simulink model "BatteryPack"  (R2023b)
settings: Solver=VariableStepAuto  StartTime=0.0  StopTime=10.0  RelTol=1e-3
InitFcn:
  | eta=0.992943452611046;
  | Q=5.134436834270520;
  | Qinv=1/Q;
  | Qinv_cells=Qinv+0.01*rand(12,1);
  | delta_t=0.1;
  | delta_t_delta=4;
  | taw=2.410723815561624;
  | R0=0.011163238296886;
  | R0_cells=R0+0.001*rand(12,1);
  | R=0.002515135572506;
  | gamma=61.749752200480295;
  | M0=0.002542395121461;
  | M=0.044341699418566;
  | OCV0=[3.03083668947220,3.16996176507765,3.24654613672245,3.30462471088150,3.35178831826018,3.39207985837564,3.42754280925954,3.45930893308633,3.48845834377828,3.51506471884948,3.53941528250350,3.56229005089512,3.58347680139773,3.60345371361795,3.62204667414497,3.63945293994712,3.65555208129593,3.67025842747189,3.68283722926942,3.69256635796299,3.69934356504319,3.70421492193387,3.70864080668278,3.71251647816700,3.71676450243010,3.72076080442289,3.72459036631361,3.72852113964889,3.73262555664002,3.73679788031633,3.74085805813141,3.74504293170943,3.74937151420852,3.75360503345497,3.75808554938499,3.76253512812700,3.76686713224277,3.77129741354356,3.77568299945893,3.78010899552110,3.78432597237866,3.78866667245794,3.79282973590265,3.79699149175738,3.80102646886227,3.80486901671467,3.80859160652083,3.81234290326678,3.81578374146922,3.81901029060391,3.82246264968075,3.82565270541301,3.82878492908885,3.83182846251259,3.83504605065465,3.83817152994830,3.84120926637331,3.84427045104513,3.84745505461551,3.85048527227548,3.85338258086535,3.85633375142700,3.85903736950342,3.86183294078638,3.86426909473005,3.86668409269911,3.86884960464201,3.87075062579497,3.87260151166861,3.87419873493045,3.87590354579771,3.87742660309802,3.87888623494178,3.88013778482297,3.88172955555187,3.88298517380087,3.88445139467736,3.88588841874555,3.88718906620625,3.88865483707461,3.89034900018679,3.89177308296385,3.89345014882802,3.89492324307466,3.89656804158261,3.89814831273987,3.89970800088682,3.90138268502894,3.90325919869100,3.90466035566401,3.90650715226313,3.90818394205928,3.90991726595604,3.91178869314647,3.91353048350435,3.91535717290223,3.91722943087205,3.91902077537227,3.92094773764149,3.92272669049051,3.92480210727778,3.92665898861166,3.92855163124444,3.93049425931182,3.93233822864100,3.93413808807444,3.93586787406902,3.93781878301823,3.93970352375448,3.94141217835583,3.94337738846496,3.94524781610469,3.94705512196599,3.94889596931986,3.95072813117993,3.95268786149774,3.95437483545637,3.95614043217004,3.95813802002780,3.95988737276266,3.96180145819164,3.96333094922522,3.96513598465409,3.96688905019200,3.96847526303094,3.97032227257873,3.97189764460202,3.97357890138617,3.97507568580842,3.97666308363629,3.97834004990894,3.97972757215233,3.98134719919954,3.98282452838428,3.98434240750033,3.98579080664983,3.98712095624815,3.98848186479248,3.99005169119157,3.99140961007081,3.99272279272243,3.99405266719970,3.99553040552875,3.99686295933407,3.99826042332052,3.99959085613132,4.00118770124588,4.00258756750194,4.00410831223298,4.00564378913664,4.00733579962478,4.00874100440808,4.01049664802522,4.01229894715480,4.01403904622199,4.01578258632489,4.01777261837808,4.01971351876421,4.02181419747090,4.02405411757281,4.02634132187682,4.02844966043338,4.03074821161091,4.03287252710406,4.03519979075052,4.03714724603729,4.03920059502787,4.04119005170582,4.04311251958802,4.04485629277420,4.04687276700581,4.04856655229106,4.05028282064349,4.05188790780758,4.05367115501827,4.05540888556017,4.05715082708000,4.05891707849673,4.06058066558082,4.06255984784218,4.06443355862160,4.06646437679668,4.06828978114252,4.07040446117501,4.07260180541029,4.07472443659757,4.07695226365058,4.07952388568996,4.08211497603818,4.08494517654941,4.08785760361077,4.09108975271414,4.09441257923899,4.09808703497329,4.10213358582538,4.10639223642507,4.11114147862302,4.11656968526475,4.12276605724301,4.13028542232852,4.14480757713318];
  | OCVrel=[-0.000420362949371303,-0.000578339102606499,-0.000548212633161139,-0.000532050376255593,-0.000513855468461292,-0.000495687320522634,-0.000487643250941371,-0.000470920985950642,-0.000461928451583620,-0.000448574992511236,-0.000430345291794665,-0.000415864789930715,-0.000403503275736067,-0.000392608506451838,-0.000381149699535297,-0.000369136346590911,-0.000348156127830507,-0.000324184515919599,-0.000280229092973681,-0.000201932662233446,-0.000110744926726894,-3.79084757376537e-05,7.34820416665105e-08,1.98249344364182e-05,1.89028531032423e-05,1.52778169972465e-05,1.34924868477160e-05,9.23542420261725e-06,-1.46245586440975e-06,-1.45311365618779e-05,-2.47366010229282e-05,-3.53430095058658e-05,-4.35761509840300e-05,-4.95443607046995e-05,-5.59569418266839e-05,-5.71405250985218e-05,-5.58628466608733e-05,-5.23710248925624e-05,-5.22024906444821e-05,-5.10066281299635e-05,-4.60070072284917e-05,-4.39210588487260e-05,-4.17087376582674e-05,-3.79965319780425e-05,-3.52883378328963e-05,-2.96358522826692e-05,-1.93487210265394e-05,-1.76654799578108e-05,-1.10481636980021e-05,-6.29033346947879e-06,-6.43729682754031e-06,-8.99082338466702e-06,-5.97476480532998e-06,-4.62198779734926e-06,-8.45626888598137e-06,-3.55310580626464e-06,1.21105779784145e-06,3.23270957394308e-06,4.65975925632772e-06,6.06047576788568e-06,1.06741421249725e-05,1.27740668978125e-05,1.58322240631086e-05,1.58226143080902e-05,1.77356396535024e-05,1.67297263145319e-05,2.20422014608934e-05,3.24455524629346e-05,4.53671310943400e-05,6.36631547519500e-05,7.65783816690908e-05,9.78737779086299e-05,0.000118072210378981,0.000145052733908454,0.000159053964033644,0.000178615115542580,0.000192951944721033,0.000203745870809340,0.000215887472157157,0.000217389449254637,0.000214080259255523,0.000217368801393146,0.000210680488604522,0.000216791472310507,0.000210807141665482,0.000206892775031066,0.000209889448971827,0.000206480366569060,0.000197477832361696,0.000201878205171392,0.000195991461516702,0.000193299624131949,0.000189225295900371,0.000183015755985024,0.000181030375137689,0.000179058026812520,0.000172630244233569,0.000169739554492468,0.000168470860940041,0.000165673583835095,0.000158761613569570,0.000158310548246597,0.000160768730786868,0.000159274891317150,0.000163654237071923,0.000165646854650985,0.000171009006229332,0.000172960872040281,0.000174059186593325,0.000184792008315373,0.000185457536514424,0.000188497928404933,0.000193540560057086,0.000201967121634793,0.000208651810099923,0.000210203310502306,0.000221327742354831,0.000226934798568295,0.000229022527795167,0.000235980838038274,0.000237393722897026,0.000251416377586933,0.000255669183930939,0.000259582507624291,0.000271756110286130,0.000271428141354407,0.000280338423121521,0.000282159563486788,0.000293698306662556,0.000294690382734668,0.000296368480075595,0.000305852381154249,0.000305547730725772,0.000310124564075650,0.000308910141248888,0.000310910207998593,0.000317136879477080,0.000319966110029179,0.000317781933009713,0.000319714895363342,0.000323633211007860,0.000324670146330631,0.000321258389806546,0.000325090635960723,0.000325756317802870,0.000329299487485483,0.000323022114762843,0.000329687741218402,0.000331335077114761,0.000334366863810491,0.000334190313302610,0.000348244516476559,0.000353619969496185,0.000370645612717080,0.000387424759796793,0.000412712601107454,0.000432980002313212,0.000458081645703528,0.000475316126710853,0.000488710969037302,0.000490229811285922,0.000496997034255361,0.000490732502998424,0.000485413024014050,0.000470031399074122,0.000464225038785084,0.000453594366571016,0.000442947689735187,0.000432361194051228,0.000426870028472560,0.000412534978795853,0.000404144406879032,0.000399500637103100,0.000395361789641937,0.000391903989806764,0.000388094198725783,0.000384493593513828,0.000380890719331740,0.000381944387481867,0.000375725748044827,0.000377689116895975,0.000371263292977880,0.000375401761542324,0.000371961214504098,0.000372140497419301,0.000376623010739057,0.000379713082469440,0.000373305112977953,0.000376271071938692,0.000374048457576144,0.000373866132643822,0.000368451986163444,0.000366513632840686,0.000361449855405437,0.000355758001511034,0.000351852945592445,0.000340424192937049,0.000323803410913197,0.000299570003101876,0.000255297108741397,9.12380218506306e-05];
  | soc_values=[0,0.00500000000000000,0.0100000000000000,0.0150000000000000,0.0200000000000000,0.0250000000000000,0.0300000000000000,0.0350000000000000,0.0400000000000000,0.0450000000000000,0.0500000000000000,0.0550000000000000,0.0600000000000000,0.0650000000000000,0.0700000000000000,0.0750000000000000,0.0800000000000000,0.0850000000000000,0.0900000000000000,0.0950000000000000,0.100000000000000,0.105000000000000,0.110000000000000,0.115000000000000,0.120000000000000,0.125000000000000,0.130000000000000,0.135000000000000,0.140000000000000,0.145000000000000,0.150000000000000,0.155000000000000,0.160000000000000,0.165000000000000,0.170000000000000,0.175000000000000,0.180000000000000,0.185000000000000,0.190000000000000,0.195000000000000,0.200000000000000,0.205000000000000,0.210000000000000,0.215000000000000,0.220000000000000,0.225000000000000,0.230000000000000,0.235000000000000,0.240000000000000,0.245000000000000,0.250000000000000,0.255000000000000,0.260000000000000,0.265000000000000,0.270000000000000,0.275000000000000,0.280000000000000,0.285000000000000,0.290000000000000,0.295000000000000,0.300000000000000,0.305000000000000,0.310000000000000,0.315000000000000,0.320000000000000,0.325000000000000,0.330000000000000,0.335000000000000,0.340000000000000,0.345000000000000,0.350000000000000,0.355000000000000,0.360000000000000,0.365000000000000,0.370000000000000,0.375000000000000,0.380000000000000,0.385000000000000,0.390000000000000,0.395000000000000,0.400000000000000,0.405000000000000,0.410000000000000,0.415000000000000,0.420000000000000,0.425000000000000,0.430000000000000,0.435000000000000,0.440000000000000,0.445000000000000,0.450000000000000,0.455000000000000,0.460000000000000,0.465000000000000,0.470000000000000,0.475000000000000,0.480000000000000,0.485000000000000,0.490000000000000,0.495000000000000,0.500000000000000,0.505000000000000,0.510000000000000,0.515000000000000,0.520000000000000,0.525000000000000,0.530000000000000,0.535000000000000,0.540000000000000,0.545000000000000,0.550000000000000,0.555000000000000,0.560000000000000,0.565000000000000,0.570000000000000,0.575000000000000,0.580000000000000,0.585000000000000,0.590000000000000,0.595000000000000,0.600000000000000,0.605000000000000,0.610000000000000,0.615000000000000,0.620000000000000,0.625000000000000,0.630000000000000,0.635000000000000,0.640000000000000,0.645000000000000,0.650000000000000,0.655000000000000,0.660000000000000,0.665000000000000,0.670000000000000,0.675000000000000,0.680000000000000,0.685000000000000,0.690000000000000,0.695000000000000,0.700000000000000,0.705000000000000,0.710000000000000,0.715000000000000,0.720000000000000,0.725000000000000,0.730000000000000,0.735000000000000,0.740000000000000,0.745000000000000,0.750000000000000,0.755000000000000,0.760000000000000,0.765000000000000,0.770000000000000,0.775000000000000,0.780000000000000,0.785000000000000,0.790000000000000,0.795000000000000,0.800000000000000,0.805000000000000,0.810000000000000,0.815000000000000,0.820000000000000,0.825000000000000,0.830000000000000,0.835000000000000,0.840000000000000,0.845000000000000,0.850000000000000,0.855000000000000,0.860000000000000,0.865000000000000,0.870000000000000,0.875000000000000,0.880000000000000,0.885000000000000,0.890000000000000,0.895000000000000,0.900000000000000,0.905000000000000,0.910000000000000,0.915000000000000,0.920000000000000,0.925000000000000,0.930000000000000,0.935000000000000,0.940000000000000,0.945000000000000,0.950000000000000,0.955000000000000,0.960000000000000,0.965000000000000,0.970000000000000,0.975000000000000,0.980000000000000,0.985000000000000,0.990000000000000,0.995000000000000,1];
  | OCV_values=OCV0+25*OCVrel;
  | dZ = soc_values(2) - soc_values(1); % Find spacing of SOC vector
  | dUdZ = diff(OCV_values)/dZ; % Scaled forward finite difference
  | dOCV = ([dUdZ(1) dUdZ] + [dUdZ dUdZ(end)])/2; % Avg of fwd/bkwd diffs
  | SigmaX0 = diag([1e-3 1e-3 1e-2]); % uncertainty of initial state
  | sigmaV = 2e-1; % uncertainty of voltage sensor, output equation
  | sigmaW = 1e1; % uncertainty of current sensor, state equation
  | vbar=0;
  | w_bar=0;
  | nR=0.004;
  | nQ=0.05;
  | ek=0.01;
  | Vmax=4.2;
  | Vmin=2.7;
  | Imax=2*Q;
  | Standby=0;
  | Charging=1;
  | Discharging=2;
  | load('BattCrntDrvCycle.mat');
undefined symbols (not defined in the file): AUX0_OV, AUX1_OV, AUX2_OV, AUX3_OV, AUX4_OV, NCHAN
libraries: fl_lib x130, nesl_utility x88, simulink x53, ee_lib x37, batt_lib x36, eeGeneralControl x21, hdlsllib x9
(part 1 of 10)
settings Model: Creator=Alkhouly  LastModifiedBy=Alkhouly

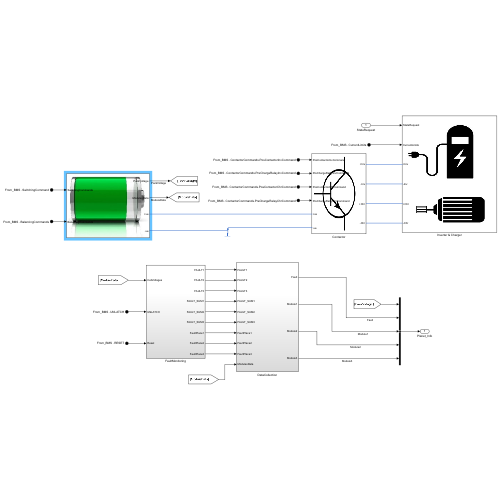
[thumbnail: Simulink's stored preview of the top-level diagram]
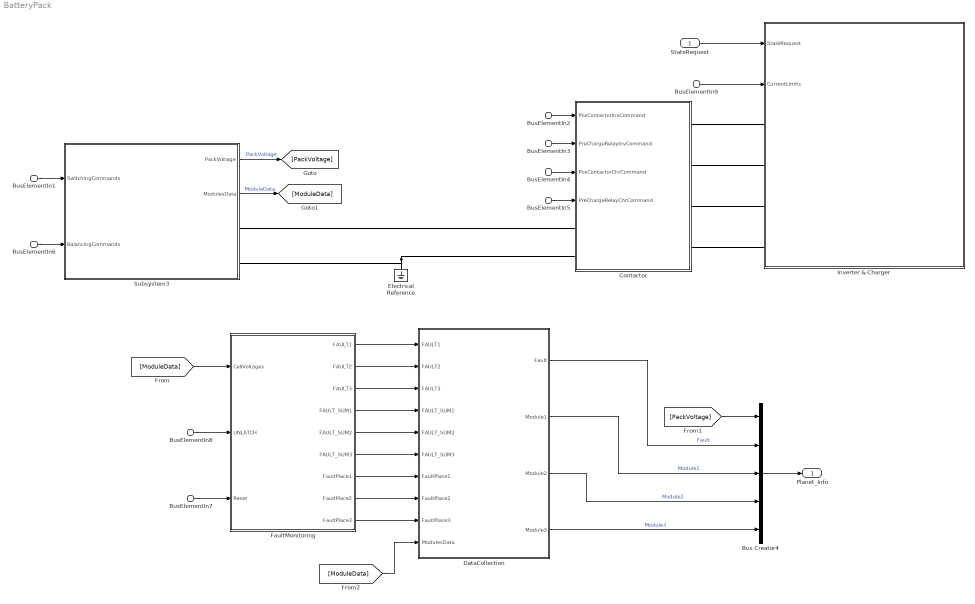
== system BatteryPack ==
  StateRequest : Inport
  BusElementIn2 : Inport  Port=2  PortName=From_BMS  Element=ContactorCommands.PosContactorInvCommand
  BusElementIn3 : Inport  Port=2  PortName=From_BMS  Element=ContactorCommands.PreChargeRelayInvCommand
  BusElementIn4 : Inport  Port=2  PortName=From_BMS  Element=ContactorCommands.PosContactorChrCommand
  BusElementIn5 : Inport  Port=2  PortName=From_BMS  Element=ContactorCommands.PreChargeRelayChrCommand
  BusElementIn1 : Inport  Port=2  PortName=From_BMS  Element=SwitchingCommand
  BusElementIn8 : Inport  Port=2  PortName=From_BMS  Element=UNLATCH
  BusElementIn7 : Inport  Port=2  PortName=From_BMS  Element=RESET
  BusElementIn6 : Inport  Port=2  PortName=From_BMS  Element=BalancingCommands
  BusElementIn9 : Inport  Port=2  PortName=From_BMS  Element=CurrentLimits
  Bus Creator4 : BusCreator  Inputs=5
  Contactor : Subsystem
      mask Display: image('PowerElectronics.jpg');
  DataCollection : Subsystem
  Electrical Reference : fl_lib/Electrical/Electrical Elements/Electrical Reference
  FaultMonitoring : Subsystem
  Inverter & Charger : Subsystem
      mask Display: image('Charger_Load3.jpg');
  Subsystem3 : Subsystem
      mask Display: image('Plant_Battery.jpg');
  Planet_Info : Outport
  wires:
  StateRequest/1 -> Inverter & Charger/1(StateRequest)
  Subsystem3/1(PackVoltage) -> [PackVoltage]  "PackVoltage"
  Subsystem3/2(ModulesData) -> [ModuleData]  "ModuleData"
  [ModuleData] -> FaultMonitoring/1(CellVoltages)
  [PackVoltage] -> Bus Creator4/1
  BusElementIn2/1 -> Contactor/1(PosContactorInvCommand)
  BusElementIn3/1 -> Contactor/2(PreChargeRelayInvCommand)
  BusElementIn4/1 -> Contactor/3(PosContactorChrCommand)
  BusElementIn5/1 -> Contactor/4(PreChargeRelayChrCommand)
  BusElementIn1/1 -> Subsystem3/1(SwitchingCommands)
  BusElementIn6/1 -> Subsystem3/2(BalancingCommands)
  BusElementIn7/1 -> FaultMonitoring/3(Reset)
  BusElementIn8/1 -> FaultMonitoring/2(UNLATCH)
  BusElementIn9/1 -> Inverter & Charger/2(CurrentLimits)
  FaultMonitoring/1(FAULT1) -> DataCollection/1(FAULT1)
  FaultMonitoring/2(FAULT2) -> DataCollection/2(FAULT2)
  FaultMonitoring/3(FAULT3) -> DataCollection/3(FAULT3)
  FaultMonitoring/4(FAULT_SUM1) -> DataCollection/4(FAULT_SUM1)
  FaultMonitoring/5(FAULT_SUM2) -> DataCollection/5(FAULT_SUM2)
  FaultMonitoring/6(FAULT_SUM3) -> DataCollection/6(FAULT_SUM3)
  FaultMonitoring/7(FaultPlace1) -> DataCollection/7(FaultPlace1)
  FaultMonitoring/8(FaultPlace2) -> DataCollection/8(FaultPlace2)
  FaultMonitoring/9(FaultPlace3) -> DataCollection/9(FaultPlace3)
  [ModuleData] -> DataCollection/10(ModulesData)
  DataCollection/1(Fault) -> Bus Creator4/2  "Fault"
  DataCollection/2(Module1) -> Bus Creator4/3  "Module1"
  DataCollection/3(Module2) -> Bus Creator4/4  "Module2"
  DataCollection/4(Module3) -> Bus Creator4/5  "Module3"
  Bus Creator4/1 -> Planet_Info/1
  connections:
  Subsystem3/RConn1 -- Contactor/LConn1
  Contactor/RConn3 -- Inverter & Charger/LConn3
  Contactor/RConn2 -- Inverter & Charger/LConn2
  Contactor/RConn4 -- Inverter & Charger/LConn4
  Contactor/RConn1 -- Inverter & Charger/LConn1
  Subsystem3/RConn2 -- Electrical Reference/LConn1 -- Contactor/LConn2

== system BatteryPack/Contactor ==
  PosContactorInvCommand : Inport
  PreChargeRelayInvCommand : Inport  Port=2
  PosContactorChrCommand : Inport  Port=3
  PreChargeRelayChrCommand : Inport  Port=4
  Capacitor : fl_lib/Electrical/Electrical Elements/Capacitor  c=10000 uF  r=1e-6 Ohm  g=0 1/Ohm  i_specify=off  i_priority=None  i=0 A  i_nominal_specify=off  i_nominal_unit=A  i_nominal_value=1  v_specify=off  v_priority=None  v=0 V  v_nominal_specify=off  v_nominal_unit=V  v_nominal_value=1  vc_specify=off  vc_priority=High  vc=0 V  vc_nominal_specify=off  vc_nominal_unit=V  vc_nominal_value=1
  Capacitor1 : fl_lib/Electrical/Electrical Elements/Capacitor  c=10000 uF  r=1e-6 Ohm  g=0 1/Ohm  i_specify=off  i_priority=None  i=0 A  i_nominal_specify=off  i_nominal_unit=A  i_nominal_value=1  v_specify=off  v_priority=None  v=0 V  v_nominal_specify=off  v_nominal_unit=V  v_nominal_value=1  vc_specify=off  vc_priority=High  vc=0 V  vc_nominal_specify=off  vc_nominal_unit=V  vc_nominal_value=1
  Data Type Conversion{,1,3..4} (4 alike) : DataTypeConversion  SaturateOnIntegerOverflow=off  RndMeth=Floor
  Resistor : fl_lib/Electrical/Electrical Elements/Resistor  R=20 Ohm  i_specify=off  i_priority=None  i=0 A  i_nominal_specify=off  i_nominal_unit=A  i_nominal_value=1  v_specify=off  v_priority=None  v=0 V  v_nominal_specify=off  v_nominal_unit=V  v_nominal_value=1
  Resistor1 : fl_lib/Electrical/Electrical Elements/Resistor  R=20 Ohm  i_specify=off  i_priority=None  i=0 A  i_nominal_specify=off  i_nominal_unit=A  i_nominal_value=1  v_specify=off  v_priority=None  v=0 V  v_nominal_specify=off  v_nominal_unit=V  v_nominal_value=1
  Simulink-PS Converter{,1,3..4} (4 alike) : nesl_utility/Simulink-PS Converter  PhysicalDomain=network_engine_domain  SubClassName=ps_input  LeftPortType=input  RightPortType=output  PseudoPeriodic=off  Frequencies=[]  NoiseDistribution=none  NoiseParameters=[]  Unit=1  AffineConversion=off  FilteringAndDerivatives=provide  SimscapeFilterOrder=1  InputFilterTimeConstant=0.001  UdotUserProvided=0
  Switch{,2..4} (4 alike) : fl_lib/Electrical/Electrical Elements/Switch  R_closed=0.01 Ohm  G_open=1e-8 1/Ohm  Threshold=0.5  i_specify=off  i_priority=None  i=0 A  i_nominal_specify=off  i_nominal_unit=A  i_nominal_value=1  v_specify=off  v_priority=None  v=0 V  v_nominal_specify=off  v_nominal_unit=V  v_nominal_value=1
  +ve : PMIOPort  Side=Left
  -ve : PMIOPort  Port=2  Side=Left
  +Inv : PMIOPort  Port=3  Side=Right
  -Inv : PMIOPort  Port=4  Side=Right
  +Chr : PMIOPort  Port=5  Side=Right
  -Chr : PMIOPort  Port=6  Side=Right
  wires:
  PosContactorInvCommand/1 -> Data Type Conversion/1
  PreChargeRelayInvCommand/1 -> Data Type Conversion1/1
  PosContactorChrCommand/1 -> Data Type Conversion3/1
  PreChargeRelayChrCommand/1 -> Data Type Conversion4/1
  Data Type Conversion/1 -> Simulink-PS Converter/1
  Data Type Conversion1/1 -> Simulink-PS Converter1/1
  Data Type Conversion3/1 -> Simulink-PS Converter3/1
  Data Type Conversion4/1 -> Simulink-PS Converter4/1
  connections:
  Switch2/RConn2 -- Switch4/RConn2 -- Switch/RConn2 -- +ve/RConn1 -- Switch3/RConn2
  Resistor/LConn1 -- Switch4/LConn1
  Resistor1/LConn1 -- Switch3/LConn1
  Switch/LConn1 -- Capacitor1/LConn1 -- +Inv/RConn1 -- Resistor/RConn1
  Switch2/LConn1 -- Capacitor/LConn1 -- +Chr/RConn1 -- Resistor1/RConn1
  -ve/RConn1 -- -Inv/RConn1 -- Capacitor1/RConn1 -- Capacitor/RConn1 -- -Chr/RConn1
  Simulink-PS Converter/RConn1 -- Switch/RConn1
  Simulink-PS Converter1/RConn1 -- Switch4/RConn1
  Simulink-PS Converter3/RConn1 -- Switch2/RConn1
  Simulink-PS Converter4/RConn1 -- Switch3/RConn1

== system BatteryPack/DataCollection ==
  FAULT1 : Inport
  FAULT2 : Inport  Port=2
  FAULT3 : Inport  Port=3
  FAULT_SUM1 : Inport  Port=4
  FAULT_SUM2 : Inport  Port=5
  FAULT_SUM3 : Inport  Port=6
  FaultPlace1 : Inport  Port=7
  FaultPlace2 : Inport  Port=8
  FaultPlace3 : Inport  Port=9
  ModulesData : Inport  Port=10
  Bus Selector : BusSelector  OutputSignals=Module1,Module2,Module3
  OR : Logic  Operator=OR  Inputs=3  AllPortsSameDT=off  OutDataTypeStr=boolean
  Fault : Outport
  Bus Element Out : Outport  Port=2  PortName=Module1  Element=FAULT1
  BusElementOut : Outport  Port=2  PortName=Module1  Element=FAULT_SUM1
  BusElementOut1 : Outport  Port=2  PortName=Module1  Element=FaultPlace1
  BusElementOut2 : Outport  Port=2  PortName=Module1  Element=ModuleData1
  Bus Element Out1 : Outport  Port=3  PortName=Module2  Element=FAULT2
  BusElementOut3 : Outport  Port=3  PortName=Module2  Element=FAULT_SUM2
  BusElementOut4 : Outport  Port=3  PortName=Module2  Element=FaultPlace2
  BusElementOut5 : Outport  Port=3  PortName=Module2  Element=ModuleData2
  Bus Element Out2 : Outport  Port=4  PortName=Module3  Element=FAULT3
  BusElementOut6 : Outport  Port=4  PortName=Module3  Element=FAULT_SUM3
  BusElementOut7 : Outport  Port=4  PortName=Module3  Element=FaultPlace3
  BusElementOut8 : Outport  Port=4  PortName=Module3  Element=ModuleData3
  wires:
  FAULT1/1 -> OR/1, Bus Element Out/1
  FAULT_SUM1/1 -> BusElementOut/1
  FaultPlace1/1 -> BusElementOut1/1
  ModulesData/1 -> Bus Selector/1
  Bus Selector/1 -> BusElementOut2/1  "<Module1>"
  Bus Selector/2 -> BusElementOut5/1  "<Module2>"
  FaultPlace2/1 -> BusElementOut4/1
  FAULT2/1 -> OR/2, Bus Element Out1/1
  FAULT_SUM2/1 -> BusElementOut3/1
  FAULT3/1 -> OR/3, Bus Element Out2/1
  FAULT_SUM3/1 -> BusElementOut6/1
  FaultPlace3/1 -> BusElementOut7/1
  Bus Selector/3 -> BusElementOut8/1  "<Module3>"
  OR/1 -> Fault/1

== system BatteryPack/FaultMonitoring ==
  note: مهم ركز الlatch هو الاصل
  note: الIC لسه فيها secondary protector
  note: 3) ضبض الFO_CTRL بحيث نعمل enable للfaults
  note: 2)ما عنديش غير protection لل
      | discahrge لو عاوز تجيب الcharge لازم تجيب sensor بالعكس
  note: 1) أنا حاطط 3 sensor currentوكل واحد ليه قرائته على slave فهيتقارن الثلاثة مع بعض
  note: ممكن تاخد الfaultMonitering state machine من project 2019
  note: احنا بنعمل model للslave هنا بنحاكي بس الfault فأنا شايف إن بالنسبة للcurrent مادام كده كده هدخله على slave خليه ياخد الthreshold بتاعه من slave
  BusElementIn1 : Inport  PortName=CellVoltages  Element=Module1.CellVoltages1
  BusElementIn : Inport  PortName=CellVoltages  Element=Module1.CurrentModule1
  BusElementIn2 : Inport  PortName=CellVoltages  Element=Module2.CellVoltages2
  BusElementIn3 : Inport  PortName=CellVoltages  Element=Module2.CurrentModule2
  BusElementIn4 : Inport  PortName=CellVoltages  Element=Module3.CellVoltages3
  BusElementIn5 : Inport  PortName=CellVoltages  Element=Module3.CurrentModule3
  In Bus Element : Inport  Port=2  PortName=UNLATCH  Element=UNLATCH1
  BusElementIn6 : Inport  Port=2  PortName=UNLATCH  Element=UNLATCH2
  BusElementIn7 : Inport  Port=2  PortName=UNLATCH  Element=UNLATCH3
  In Bus Element1 : Inport  Port=3  PortName=Reset  Element=RESET1
  BusElementIn8 : Inport  Port=3  PortName=Reset  Element=RESET2
  BusElementIn9 : Inport  Port=3  PortName=Reset  Element=RESET3
  Subsystem1 : Subsystem
  Subsystem2 : Subsystem
  Subsystem3 : Subsystem
  FAULT1 : Outport
  FAULT2 : Outport  Port=2
  FAULT3 : Outport  Port=3
  FAULT_SUM1 : Outport  Port=4
  FAULT_SUM2 : Outport  Port=5
  FAULT_SUM3 : Outport  Port=6
  FaultPlace1 : Outport  Port=7
  FaultPlace2 : Outport  Port=8
  FaultPlace3 : Outport  Port=9
  wires:
  Subsystem1/2(FAULT_SUM) -> FAULT_SUM1/1
  Subsystem1/1(FAULT) -> FAULT1/1
  Subsystem1/3(FaultPlace) -> FaultPlace1/1
  BusElementIn1/1 -> Subsystem1/1(CellVoltages)
  BusElementIn/1 -> Subsystem1/2(ModuleCurrent)
  BusElementIn2/1 -> Subsystem2/1(CellVoltages)
  BusElementIn3/1 -> Subsystem2/2(ModuleCurrent)
  BusElementIn4/1 -> Subsystem3/1(CellVoltages)
  BusElementIn5/1 -> Subsystem3/2(ModuleCurrent)
  Subsystem2/1(FAULT) -> FAULT2/1
  Subsystem3/1(FAULT) -> FAULT3/1
  Subsystem2/2(FAULT_SUM) -> FAULT_SUM2/1
  Subsystem3/2(FAULT_SUM) -> FAULT_SUM3/1
  Subsystem2/3(FaultPlace) -> FaultPlace2/1
  Subsystem3/3(FaultPlace) -> FaultPlace3/1
  In Bus Element/1 -> Subsystem1/3(UNLATCH)
  BusElementIn6/1 -> Subsystem2/3(UNLATCH)
  BusElementIn7/1 -> Subsystem3/3(UNLATCH)
  In Bus Element1/1 -> Subsystem1/4(Reset)
  BusElementIn8/1 -> Subsystem2/4(Reset)
  BusElementIn9/1 -> Subsystem3/4(Reset)

== system BatteryPack/Inverter & Charger ==
  StateRequest : Inport
  CurrentLimits : Inport  Port=2
  Charger : Subsystem
  Data Type Conversion : DataTypeConversion  OutDataTypeStr=uint8  SaturateOnIntegerOverflow=off  RndMeth=Floor
  Inverter : Subsystem
  +Inv : PMIOPort  Side=Left
  -Inv : PMIOPort  Port=2  Side=Left
  +Chr : PMIOPort  Port=3  Side=Left
  -Chr : PMIOPort  Port=4  Side=Left
  wires:
  Data Type Conversion/1 -> Inverter/1(StateRequest), Charger/1(StateRequest)
  StateRequest/1 -> Data Type Conversion/1
  CurrentLimits/1 -> Inverter/2(current limits)
  connections:
  +Chr/RConn1 -- Charger/LConn1
  -Chr/RConn1 -- Charger/LConn2
  +Inv/RConn1 -- Inverter/LConn1
  -Inv/RConn1 -- Inverter/LConn2

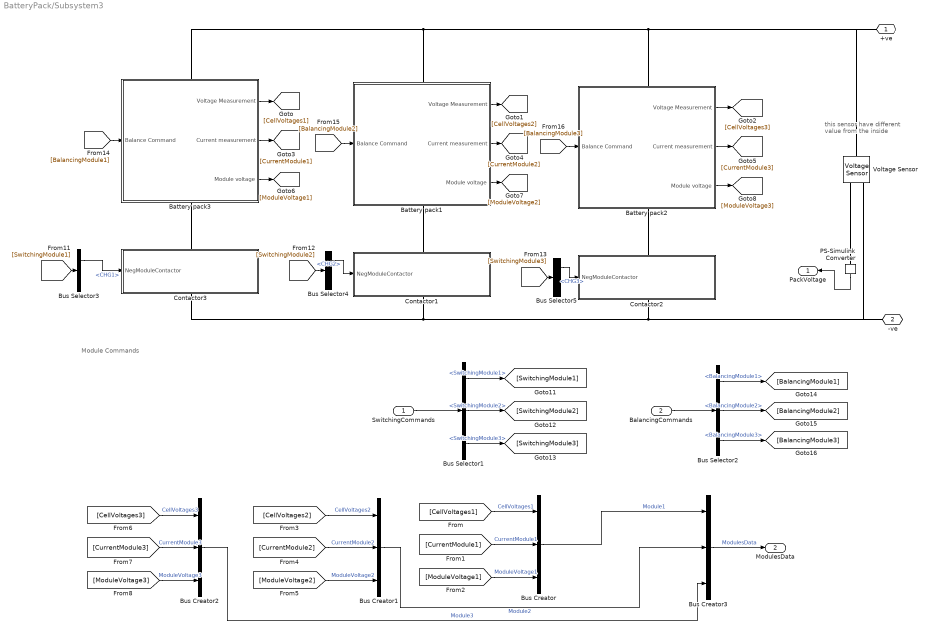
== system BatteryPack/Subsystem3 ==
  note: Module Commands
  note: this sensor have
      | different value
      | from the inside
  SwitchingCommands : Inport
  BalancingCommands : Inport  Port=2
  Battery pack1 : Subsystem
      settings: PortSchema="{\"entries\":[{\"content\":{\"sides\":[{\"content\":{\"connectorIds\":[\"In1\"]},\"type\":\"ConnectorPlacement.EquallySpacedRectSide\",\"uuid\":\"a3c89816-d530-4a3a-b1ff-efc55dfdad15\"},{\"content\":{\"connectorIds\":[\"Out1\",\"Out2\",\"Out3\"],\"side\":\"RIGHT\"},\"type\":\"ConnectorPlacement.EquallySpacedRectSide\",\"uuid\":\"1a53a330-7246-4d3e-a25a-32a75c8e4af7\"},{\"content\":{\"connectorIds\":[\"LConn1\"],\"side\":\"TOP\"},\"type\":\"ConnectorPlacement.EquallySpacedRectSide\",\"uuid\":\"93dc65ad-4fd8-4dcb-adf6-f8dc2532677e\"},{\"content\":{\"connectorIds\":[\"RConn1\"],\"side\":\"BOTTOM\"},\"type\":\"ConnectorPlacement.EquallySpacedRectSide\",\"uuid\":\"d7eeecb4-f41c-40a7-b457-1be4721ba6e4\"}]},\"type\":\"ConnectorPlacement.EquallySpacedConnector\",\"uuid\":\"2fea9a10-0d3b-4763-9a99-4cd5d739b1cd\"}],\"packageUris\":[\"http://schema.mathworks.com/mf0/Connector/R2020b\"],\"version\":\"1.0\"}"
  Battery pack2 : Subsystem
      settings: PortSchema="{\"entries\":[{\"content\":{\"sides\":[{\"content\":{\"connectorIds\":[\"In1\"]},\"type\":\"ConnectorPlacement.EquallySpacedRectSide\",\"uuid\":\"a3c89816-d530-4a3a-b1ff-efc55dfdad15\"},{\"content\":{\"connectorIds\":[\"Out1\",\"Out2\",\"Out3\"],\"side\":\"RIGHT\"},\"type\":\"ConnectorPlacement.EquallySpacedRectSide\",\"uuid\":\"1a53a330-7246-4d3e-a25a-32a75c8e4af7\"},{\"content\":{\"connectorIds\":[\"LConn1\"],\"side\":\"TOP\"},\"type\":\"ConnectorPlacement.EquallySpacedRectSide\",\"uuid\":\"93dc65ad-4fd8-4dcb-adf6-f8dc2532677e\"},{\"content\":{\"connectorIds\":[\"RConn1\"],\"side\":\"BOTTOM\"},\"type\":\"ConnectorPlacement.EquallySpacedRectSide\",\"uuid\":\"d7eeecb4-f41c-40a7-b457-1be4721ba6e4\"}]},\"type\":\"ConnectorPlacement.EquallySpacedConnector\",\"uuid\":\"2fea9a10-0d3b-4763-9a99-4cd5d739b1cd\"}],\"packageUris\":[\"http://schema.mathworks.com/mf0/Connector/R2020b\"],\"version\":\"1.0\"}"
  Battery pack3 : Subsystem
      settings: PortSchema="{\"entries\":[{\"content\":{\"sides\":[{\"content\":{\"connectorIds\":[\"In1\"]},\"type\":\"ConnectorPlacement.EquallySpacedRectSide\",\"uuid\":\"a3c89816-d530-4a3a-b1ff-efc55dfdad15\"},{\"content\":{\"connectorIds\":[\"Out1\",\"Out2\",\"Out3\"],\"side\":\"RIGHT\"},\"type\":\"ConnectorPlacement.EquallySpacedRectSide\",\"uuid\":\"1a53a330-7246-4d3e-a25a-32a75c8e4af7\"},{\"content\":{\"connectorIds\":[\"LConn1\"],\"side\":\"TOP\"},\"type\":\"ConnectorPlacement.EquallySpacedRectSide\",\"uuid\":\"93dc65ad-4fd8-4dcb-adf6-f8dc2532677e\"},{\"content\":{\"connectorIds\":[\"RConn1\"],\"side\":\"BOTTOM\"},\"type\":\"ConnectorPlacement.EquallySpacedRectSide\",\"uuid\":\"d7eeecb4-f41c-40a7-b457-1be4721ba6e4\"}]},\"type\":\"ConnectorPlacement.EquallySpacedConnector\",\"uuid\":\"2fea9a10-0d3b-4763-9a99-4cd5d739b1cd\"}],\"packageUris\":[\"http://schema.mathworks.com/mf0/Connector/R2020b\"],\"version\":\"1.0\"}"
  Bus Creator{,1..3} (4 alike) : BusCreator  Inputs=3
  Bus Selector1 : BusSelector  OutputSignals=SwitchingModule1,SwitchingModule2,SwitchingModule3
  Bus Selector2 : BusSelector  OutputSignals=BalancingModule1,BalancingModule2,BalancingModule3
  Bus Selector3 : BusSelector  OutputSignals=CHG1,DSG1
  Bus Selector4 : BusSelector  OutputSignals=CHG2,DSG2
  Bus Selector5 : BusSelector  OutputSignals=CHG3,DSG3
  Contactor1 : Subsystem
      settings: PortSchema="{\"entries\":[{\"content\":{\"sides\":[{\"content\":{\"connectorIds\":[\"In1\"]},\"type\":\"ConnectorPlacement.EquallySpacedRectSide\",\"uuid\":\"57c09ad0-d34a-4e87-ab13-d619afdbe30a\"},{\"content\":{\"side\":\"RIGHT\"},\"type\":\"ConnectorPlacement.EquallySpacedRectSide\",\"uuid\":\"eba1577f-d7a9-4916-8583-2b9541184966\"},{\"content\":{\"connectorIds\":[\"LConn1\"],\"side\":\"TOP\"},\"type\":\"ConnectorPlacement.EquallySpacedRectSide\",\"uuid\":\"8ce4d05b-0533-422b-ac6c-97e718f0244e\"},{\"content\":{\"connectorIds\":[\"RConn1\"],\"side\":\"BOTTOM\"},\"type\":\"ConnectorPlacement.EquallySpacedRectSide\",\"uuid\":\"abb70b3c-bced-4368-8122-6d5425d32995\"}]},\"type\":\"ConnectorPlacement.EquallySpacedConnector\",\"uuid\":\"7db92cb2-ab30-41d2-bcd4-f4c80beae55e\"}],\"packageUris\":[\"http://schema.mathworks.com/mf0/Connector/R2020b\"],\"version\":\"1.0\"}"
  Contactor2 : Subsystem
      settings: PortSchema="{\"entries\":[{\"content\":{\"sides\":[{\"content\":{\"connectorIds\":[\"In1\"]},\"type\":\"ConnectorPlacement.EquallySpacedRectSide\",\"uuid\":\"57c09ad0-d34a-4e87-ab13-d619afdbe30a\"},{\"content\":{\"side\":\"RIGHT\"},\"type\":\"ConnectorPlacement.EquallySpacedRectSide\",\"uuid\":\"eba1577f-d7a9-4916-8583-2b9541184966\"},{\"content\":{\"connectorIds\":[\"LConn1\"],\"side\":\"TOP\"},\"type\":\"ConnectorPlacement.EquallySpacedRectSide\",\"uuid\":\"8ce4d05b-0533-422b-ac6c-97e718f0244e\"},{\"content\":{\"connectorIds\":[\"RConn1\"],\"side\":\"BOTTOM\"},\"type\":\"ConnectorPlacement.EquallySpacedRectSide\",\"uuid\":\"abb70b3c-bced-4368-8122-6d5425d32995\"}]},\"type\":\"ConnectorPlacement.EquallySpacedConnector\",\"uuid\":\"7db92cb2-ab30-41d2-bcd4-f4c80beae55e\"}],\"packageUris\":[\"http://schema.mathworks.com/mf0/Connector/R2020b\"],\"version\":\"1.0\"}"
  Contactor3 : Subsystem
      settings: PortSchema="{\"entries\":[{\"content\":{\"sides\":[{\"content\":{\"connectorIds\":[\"In1\"]},\"type\":\"ConnectorPlacement.EquallySpacedRectSide\",\"uuid\":\"57c09ad0-d34a-4e87-ab13-d619afdbe30a\"},{\"content\":{\"side\":\"RIGHT\"},\"type\":\"ConnectorPlacement.EquallySpacedRectSide\",\"uuid\":\"eba1577f-d7a9-4916-8583-2b9541184966\"},{\"content\":{\"connectorIds\":[\"LConn1\"],\"side\":\"TOP\"},\"type\":\"ConnectorPlacement.EquallySpacedRectSide\",\"uuid\":\"8ce4d05b-0533-422b-ac6c-97e718f0244e\"},{\"content\":{\"connectorIds\":[\"RConn1\"],\"side\":\"BOTTOM\"},\"type\":\"ConnectorPlacement.EquallySpacedRectSide\",\"uuid\":\"abb70b3c-bced-4368-8122-6d5425d32995\"}]},\"type\":\"ConnectorPlacement.EquallySpacedConnector\",\"uuid\":\"7db92cb2-ab30-41d2-bcd4-f4c80beae55e\"}],\"packageUris\":[\"http://schema.mathworks.com/mf0/Connector/R2020b\"],\"version\":\"1.0\"}"
  PS-Simulink Converter : nesl_utility/PS-Simulink Converter  PhysicalDomain=network_engine_domain  SubClassName=ps_output  LeftPortType=input  RightPortType=output  PseudoPeriodic=off  Frequencies=[]  VectorFormat=inherit  Unit=inherit  AffineConversion=off
  Voltage Sensor : fl_lib/Electrical/Electrical Sensors/Voltage Sensor
  +ve : PMIOPort  Side=Right
  -ve : PMIOPort  Port=2  Side=Right
  PackVoltage : Outport
  ModulesData : Outport  Port=2
  wires:
  Battery pack2/1(Voltage Measurement) -> [CellVoltages3]
  [SwitchingModule1] -> Bus Selector3/1
  [BalancingModule3] -> Battery pack2/1(Balance Command)
  Battery pack1/1(Voltage Measurement) -> [CellVoltages2]
  Battery pack3/3(Module voltage) -> [ModuleVoltage1]
  Battery pack2/2(Current measurement) -> [CurrentModule3]
  Battery pack2/3(Module voltage) -> [ModuleVoltage3]
  Bus Selector5/1 -> Contactor2/1(NegModuleContactor)  "<CHG3>"
  [BalancingModule2] -> Battery pack1/1(Balance Command)
  Bus Selector4/1 -> Contactor1/1(NegModuleContactor)  "<CHG2>"
  Battery pack3/2(Current measurement) -> [CurrentModule1]
  Battery pack1/2(Current measurement) -> [CurrentModule2]
  [SwitchingModule3] -> Bus Selector5/1
  Battery pack3/1(Voltage Measurement) -> [CellVoltages1]
  Battery pack1/3(Module voltage) -> [ModuleVoltage2]
  [SwitchingModule2] -> Bus Selector4/1
  [BalancingModule1] -> Battery pack3/1(Balance Command)
  Bus Selector3/1 -> Contactor3/1(NegModuleContactor)  "<CHG1>"
  BalancingCommands/1 -> Bus Selector2/1
  Bus Selector2/3 -> [BalancingModule3]  "<BalancingModule3>"
  Bus Selector1/3 -> [SwitchingModule3]  "<SwitchingModule3>"
  Bus Selector2/2 -> [BalancingModule2]  "<BalancingModule2>"
  Bus Selector1/2 -> [SwitchingModule2]  "<SwitchingModule2>"
  SwitchingCommands/1 -> Bus Selector1/1
  Bus Selector2/1 -> [BalancingModule1]  "<BalancingModule1>"
  Bus Selector1/1 -> [SwitchingModule1]  "<SwitchingModule1>"
  Bus Creator2/1 -> Bus Creator3/3  "Module3"
  [CurrentModule1] -> Bus Creator/2  "CurrentModule1"
  [ModuleVoltage3] -> Bus Creator2/3  "ModuleVoltage3"
  Bus Creator1/1 -> Bus Creator3/2  "Module2"
  [ModuleVoltage2] -> Bus Creator1/3  "ModuleVoltage2"
  [ModuleVoltage1] -> Bus Creator/3  "ModuleVoltage1"
  [CellVoltages2] -> Bus Creator1/1  "CellVoltages2"
  [CellVoltages1] -> Bus Creator/1  "CellVoltages1"
  Bus Creator/1 -> Bus Creator3/1  "Module1"
  [CurrentModule3] -> Bus Creator2/2  "CurrentModule3"
  [CellVoltages3] -> Bus Creator2/1  "CellVoltages3"
  [CurrentModule2] -> Bus Creator1/2  "CurrentModule2"
  Bus Creator3/1 -> ModulesData/1  "ModulesData"
  PS-Simulink Converter/1 -> PackVoltage/1
  connections:
  Contactor1/LConn1 -- Battery pack1/RConn1
  Contactor3/RConn1 -- Contactor1/RConn1 -- Contactor2/RConn1 -- -ve/RConn1 -- Voltage Sensor/RConn2
  Battery pack2/LConn1 -- Voltage Sensor/LConn1 -- +ve/RConn1 -- Battery pack1/LConn1 -- Battery pack3/LConn1
  Contactor2/LConn1 -- Battery pack2/RConn1
  Battery pack3/RConn1 -- Contactor3/LConn1
  Voltage Sensor/RConn1 -- PS-Simulink Converter/LConn1

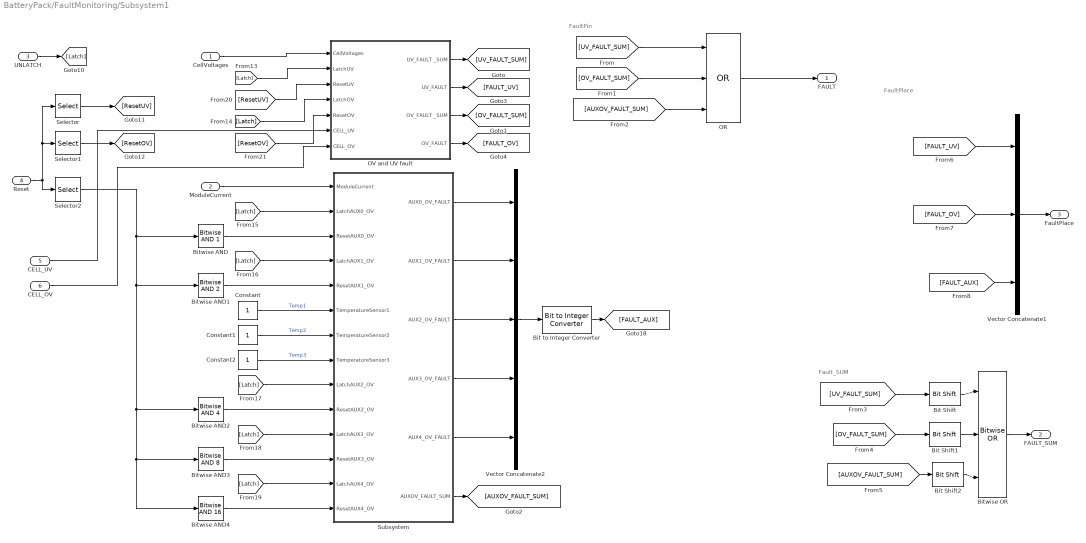
== system BatteryPack/FaultMonitoring/Subsystem1 ==
  note: FaultPlace
  note: FaultPin
  note: Fault_SUM
  CellVoltages : Inport
  ModuleCurrent : Inport  Port=2
  UNLATCH : Inport  Port=3
  Reset : Inport  Port=4
  CELL_UV : Inport  Port=5
  CELL_OV : Inport  Port=6
  Bit Shift : hdlsllib/Logic and Bit Operations/Bit Shift  mode=Shift Left Logical  N=15
  Bit Shift1 : hdlsllib/Logic and Bit Operations/Bit Shift  mode=Shift Left Logical  N=14
  Bit Shift2 : hdlsllib/Logic and Bit Operations/Bit Shift  mode=Shift Left Logical  N=12
  Bit to Integer Converter : simulink/Logic and Bit Operations/Bit to Integer Converter  nbits=5  bitOrder=LSB first  signedOutputValues=Unsigned  outDtype=Inherit via internal rule  outDtypeSigned=Inherit via internal rule
  Bitwise AND : simulink/Logic and Bit Operations/Bitwise Operator  logicop=AND  UseBitMask=on  BitMask=1  BitMaskRealWorld=Stored Integer
      settings: LibrarySourceBlock=|
      | simulink/Quick Insert/Logic and Bit
      | Operations/Bitwise AND
  Bitwise AND1 : simulink/Logic and Bit Operations/Bitwise Operator  logicop=AND  UseBitMask=on  BitMask=2  BitMaskRealWorld=Stored Integer
      settings: LibrarySourceBlock=|
      | simulink/Quick Insert/Logic and Bit
      | Operations/Bitwise AND
  Bitwise AND2 : simulink/Logic and Bit Operations/Bitwise Operator  logicop=AND  UseBitMask=on  BitMask=4  BitMaskRealWorld=Stored Integer
      settings: LibrarySourceBlock=|
      | simulink/Quick Insert/Logic and Bit
      | Operations/Bitwise AND
  Bitwise AND3 : simulink/Logic and Bit Operations/Bitwise Operator  logicop=AND  UseBitMask=on  BitMask=8  BitMaskRealWorld=Stored Integer
      settings: LibrarySourceBlock=|
      | simulink/Quick Insert/Logic and Bit
      | Operations/Bitwise AND
  Bitwise AND4 : simulink/Logic and Bit Operations/Bitwise Operator  logicop=AND  UseBitMask=on  BitMask=16  BitMaskRealWorld=Stored Integer
      settings: LibrarySourceBlock=|
      | simulink/Quick Insert/Logic and Bit
      | Operations/Bitwise AND
  Bitwise OR : simulink/Logic and Bit Operations/Bitwise Operator  logicop=OR  UseBitMask=off  NumInputPorts=3  BitMask=bin2dec('11011001')  BitMaskRealWorld=Stored Integer
      settings: LibrarySourceBlock=|
      | simulink/Quick Insert/Logic and Bit
      | Operations/Bitwise OR
  Constant : Constant
  Constant1 : Constant
  Constant2 : Constant
  OR : Logic  Operator=OR  Inputs=3  AllPortsSameDT=off  OutDataTypeStr=boolean
  OV and UV fault : Subsystem
  Selector : Selector  InputPortWidth=3  IndexOptions=Index vector (dialog)  Indices=1  OutputSizes=1
  Selector1 : Selector  InputPortWidth=3  IndexOptions=Index vector (dialog)  Indices=2  OutputSizes=1
  Selector2 : Selector  InputPortWidth=3  IndexOptions=Index vector (dialog)  Indices=3  OutputSizes=1
  Subsystem : Subsystem
  Vector Concatenate1 : Concatenate  NumInputs=3
  Vector Concatenate2 : Concatenate  NumInputs=5
  FAULT : Outport
  FAULT_SUM : Outport  Port=2
  FaultPlace : Outport  Port=3
  wires:
  Subsystem/3(AUX2_OV_FAULT) -> Vector Concatenate2/3
  [UV_FAULT_SUM] -> Bit Shift/1
  [UV_FAULT_SUM] -> OR/1
  [Latch] -> Subsystem/11(LatchAUX3_OV)
  [OV_FAULT_SUM] -> Bit Shift1/1
  [OV_FAULT_SUM] -> OR/2
  Subsystem/1(AUX0_OV_FAULT) -> Vector Concatenate2/1
  [Latch] -> Subsystem/13(LatchAUX4_OV)
  Subsystem/4(AUX3_OV_FAULT) -> Vector Concatenate2/4
  OV and UV fault/4(OV_FAULT) -> [FAULT_OV]
  OR/1 -> FAULT/1
  OV and UV fault/3(OV_FAULT _SUM) -> [OV_FAULT_SUM]
  [AUXOV_FAULT_SUM] -> Bit Shift2/1
  [AUXOV_FAULT_SUM] -> OR/3
  [ResetOV] -> OV and UV fault/5(ResetOV)
  OV and UV fault/1(UV_FAULT _SUM) -> [UV_FAULT_SUM]
  Bitwise AND3/1 -> Subsystem/12(ResetAUX3_OV)
  [Latch] -> Subsystem/9(LatchAUX2_OV)
  Subsystem/5(AUX4_OV_FAULT) -> Vector Concatenate2/5
  OV and UV fault/2(UV_FAULT) -> [FAULT_UV]
  Subsystem/6(AUXOV_FAULT_SUM) -> [AUXOV_FAULT_SUM]
  Bitwise AND/1 -> Subsystem/3(ResetAUX0_OV)
  Vector Concatenate1/1 -> FaultPlace/1
  Bitwise AND2/1 -> Subsystem/10(ResetAUX2_OV)
  [ResetUV] -> OV and UV fault/3(ResetUV)
  [FAULT_OV] -> Vector Concatenate1/2
  Bitwise OR/1 -> FAULT_SUM/1
  [Latch] -> OV and UV fault/4(LatchOV)
  [FAULT_UV] -> Vector Concatenate1/1
  [Latch] -> Subsystem/2(LatchAUX0_OV)
  Subsystem/2(AUX1_OV_FAULT) -> Vector Concatenate2/2
  [Latch] -> Subsystem/4(LatchAUX1_OV)
  Bitwise AND1/1 -> Subsystem/5(ResetAUX1_OV)
  CellVoltages/1 -> OV and UV fault/1(CellVoltages)
  ModuleCurrent/1 -> Subsystem/1(ModuleCurrent)
  UNLATCH/1 -> [Latch]
  [Latch] -> OV and UV fault/2(LatchUV)
  Selector/1 -> [ResetUV]
  Selector1/1 -> [ResetOV]
  Constant/1 -> Subsystem/6(TemperatureSensor1)  "Temp1"
  Constant1/1 -> Subsystem/7(TemperatureSensor2)  "Temp2"
  Constant2/1 -> Subsystem/8(TemperatureSensor3)  "Temp3"
  Reset/1 -> Selector1/1, Selector/1, Selector2/1
  Bitwise AND4/1 -> Subsystem/14(ResetAUX4_OV)
  Vector Concatenate2/1 -> Bit to Integer Converter/1
  Bit to Integer Converter/1 -> [FAULT_AUX]
  [FAULT_AUX] -> Vector Concatenate1/3
  Bit Shift1/1 -> Bitwise OR/2
  Bit Shift2/1 -> Bitwise OR/3
  Bit Shift/1 -> Bitwise OR/1
  Selector2/1 -> Bitwise AND/1, Bitwise AND2/1, Bitwise AND3/1, Bitwise AND4/1, Bitwise AND1/1
  CELL_UV/1 -> OV and UV fault/6(CELL_UV)
  CELL_OV/1 -> OV and UV fault/7(CELL_OV)

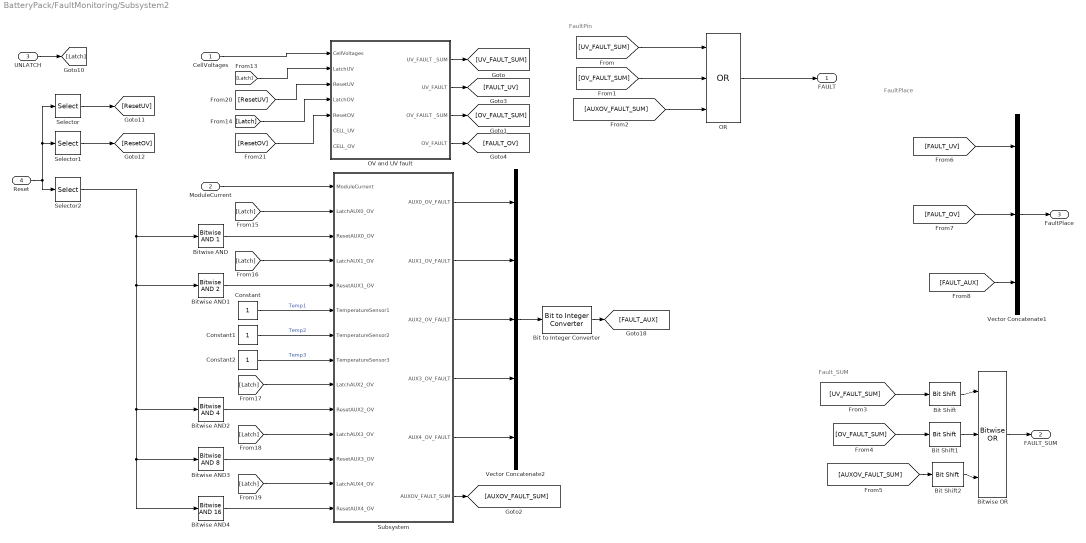
== system BatteryPack/FaultMonitoring/Subsystem2 ==
  note: FaultPlace
  note: FaultPin
  note: Fault_SUM
  CellVoltages : Inport
  ModuleCurrent : Inport  Port=2
  UNLATCH : Inport  Port=3
  Reset : Inport  Port=4
  Bit Shift : hdlsllib/Logic and Bit Operations/Bit Shift  mode=Shift Left Logical  N=15
  Bit Shift1 : hdlsllib/Logic and Bit Operations/Bit Shift  mode=Shift Left Logical  N=14
  Bit Shift2 : hdlsllib/Logic and Bit Operations/Bit Shift  mode=Shift Left Logical  N=12
  Bit to Integer Converter : simulink/Logic and Bit Operations/Bit to Integer Converter  nbits=5  bitOrder=LSB first  signedOutputValues=Unsigned  outDtype=Inherit via internal rule  outDtypeSigned=Inherit via internal rule
  Bitwise AND : simulink/Logic and Bit Operations/Bitwise Operator  logicop=AND  UseBitMask=on  BitMask=1  BitMaskRealWorld=Stored Integer
      settings: LibrarySourceBlock=|
      | simulink/Quick Insert/Logic and Bit
      | Operations/Bitwise AND
  Bitwise AND1 : simulink/Logic and Bit Operations/Bitwise Operator  logicop=AND  UseBitMask=on  BitMask=2  BitMaskRealWorld=Stored Integer
      settings: LibrarySourceBlock=|
      | simulink/Quick Insert/Logic and Bit
      | Operations/Bitwise AND
  Bitwise AND2 : simulink/Logic and Bit Operations/Bitwise Operator  logicop=AND  UseBitMask=on  BitMask=4  BitMaskRealWorld=Stored Integer
      settings: LibrarySourceBlock=|
      | simulink/Quick Insert/Logic and Bit
      | Operations/Bitwise AND
  Bitwise AND3 : simulink/Logic and Bit Operations/Bitwise Operator  logicop=AND  UseBitMask=on  BitMask=8  BitMaskRealWorld=Stored Integer
      settings: LibrarySourceBlock=|
      | simulink/Quick Insert/Logic and Bit
      | Operations/Bitwise AND
  Bitwise AND4 : simulink/Logic and Bit Operations/Bitwise Operator  logicop=AND  UseBitMask=on  BitMask=16  BitMaskRealWorld=Stored Integer
      settings: LibrarySourceBlock=|
      | simulink/Quick Insert/Logic and Bit
      | Operations/Bitwise AND
  Bitwise OR : simulink/Logic and Bit Operations/Bitwise Operator  logicop=OR  UseBitMask=off  NumInputPorts=3  BitMask=bin2dec('11011001')  BitMaskRealWorld=Stored Integer
      settings: LibrarySourceBlock=|
      | simulink/Quick Insert/Logic and Bit
      | Operations/Bitwise OR
  Constant : Constant
  Constant1 : Constant
  Constant2 : Constant
  OR : Logic  Operator=OR  Inputs=3  AllPortsSameDT=off  OutDataTypeStr=boolean
  OV and UV fault : Subsystem
  Selector : Selector  InputPortWidth=3  IndexOptions=Index vector (dialog)  Indices=1  OutputSizes=1
  Selector1 : Selector  InputPortWidth=3  IndexOptions=Index vector (dialog)  Indices=2  OutputSizes=1
  Selector2 : Selector  InputPortWidth=3  IndexOptions=Index vector (dialog)  Indices=3  OutputSizes=1
  Subsystem : Subsystem
  Vector Concatenate1 : Concatenate  NumInputs=3
  Vector Concatenate2 : Concatenate  NumInputs=5
  FAULT : Outport
  FAULT_SUM : Outport  Port=2
  FaultPlace : Outport  Port=3
  wires:
  Subsystem/3(AUX2_OV_FAULT) -> Vector Concatenate2/3
  [UV_FAULT_SUM] -> Bit Shift/1
  [UV_FAULT_SUM] -> OR/1
  [Latch] -> Subsystem/11(LatchAUX3_OV)
  [OV_FAULT_SUM] -> Bit Shift1/1
  [OV_FAULT_SUM] -> OR/2
  Subsystem/1(AUX0_OV_FAULT) -> Vector Concatenate2/1
  [Latch] -> Subsystem/13(LatchAUX4_OV)
  Subsystem/4(AUX3_OV_FAULT) -> Vector Concatenate2/4
  OV and UV fault/4(OV_FAULT) -> [FAULT_OV]
  OR/1 -> FAULT/1
  OV and UV fault/3(OV_FAULT _SUM) -> [OV_FAULT_SUM]
  [AUXOV_FAULT_SUM] -> Bit Shift2/1
  [AUXOV_FAULT_SUM] -> OR/3
  [ResetOV] -> OV and UV fault/5(ResetOV)
  OV and UV fault/1(UV_FAULT _SUM) -> [UV_FAULT_SUM]
  Bitwise AND3/1 -> Subsystem/12(ResetAUX3_OV)
  [Latch] -> Subsystem/9(LatchAUX2_OV)
  Subsystem/5(AUX4_OV_FAULT) -> Vector Concatenate2/5
  OV and UV fault/2(UV_FAULT) -> [FAULT_UV]
  Subsystem/6(AUXOV_FAULT_SUM) -> [AUXOV_FAULT_SUM]
  Bitwise AND/1 -> Subsystem/3(ResetAUX0_OV)
  Vector Concatenate1/1 -> FaultPlace/1
  Bitwise AND2/1 -> Subsystem/10(ResetAUX2_OV)
  [ResetUV] -> OV and UV fault/3(ResetUV)
  [FAULT_OV] -> Vector Concatenate1/2
  Bitwise OR/1 -> FAULT_SUM/1
  [Latch] -> OV and UV fault/4(LatchOV)
  [FAULT_UV] -> Vector Concatenate1/1
  [Latch] -> Subsystem/2(LatchAUX0_OV)
  Subsystem/2(AUX1_OV_FAULT) -> Vector Concatenate2/2
  [Latch] -> Subsystem/4(LatchAUX1_OV)
  Bitwise AND1/1 -> Subsystem/5(ResetAUX1_OV)
  CellVoltages/1 -> OV and UV fault/1(CellVoltages)
  ModuleCurrent/1 -> Subsystem/1(ModuleCurrent)
  UNLATCH/1 -> [Latch]
  [Latch] -> OV and UV fault/2(LatchUV)
  Selector/1 -> [ResetUV]
  Selector1/1 -> [ResetOV]
  Constant/1 -> Subsystem/6(TemperatureSensor1)  "Temp1"
  Constant1/1 -> Subsystem/7(TemperatureSensor2)  "Temp2"
  Constant2/1 -> Subsystem/8(TemperatureSensor3)  "Temp3"
  Reset/1 -> Selector1/1, Selector/1, Selector2/1
  Bitwise AND4/1 -> Subsystem/14(ResetAUX4_OV)
  Vector Concatenate2/1 -> Bit to Integer Converter/1
  Bit to Integer Converter/1 -> [FAULT_AUX]
  [FAULT_AUX] -> Vector Concatenate1/3
  Bit Shift1/1 -> Bitwise OR/2
  Bit Shift2/1 -> Bitwise OR/3
  Bit Shift/1 -> Bitwise OR/1
  Selector2/1 -> Bitwise AND/1, Bitwise AND2/1, Bitwise AND3/1, Bitwise AND4/1, Bitwise AND1/1

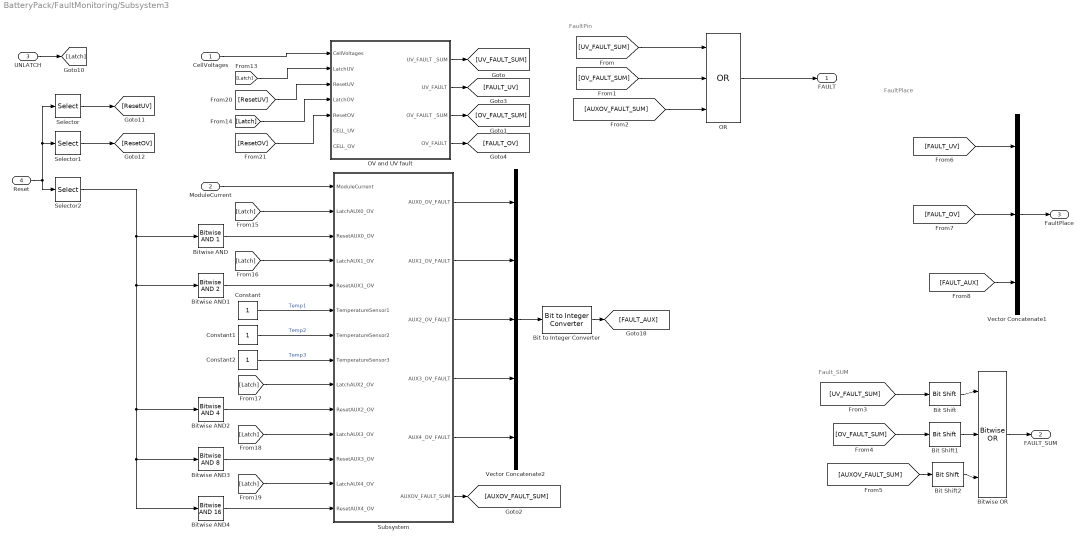
== system BatteryPack/FaultMonitoring/Subsystem3 ==
  note: FaultPlace
  note: FaultPin
  note: Fault_SUM
  CellVoltages : Inport
  ModuleCurrent : Inport  Port=2
  UNLATCH : Inport  Port=3
  Reset : Inport  Port=4
  Bit Shift : hdlsllib/Logic and Bit Operations/Bit Shift  mode=Shift Left Logical  N=15
  Bit Shift1 : hdlsllib/Logic and Bit Operations/Bit Shift  mode=Shift Left Logical  N=14
  Bit Shift2 : hdlsllib/Logic and Bit Operations/Bit Shift  mode=Shift Left Logical  N=12
  Bit to Integer Converter : simulink/Logic and Bit Operations/Bit to Integer Converter  nbits=5  bitOrder=LSB first  signedOutputValues=Unsigned  outDtype=Inherit via internal rule  outDtypeSigned=Inherit via internal rule
  Bitwise AND : simulink/Logic and Bit Operations/Bitwise Operator  logicop=AND  UseBitMask=on  BitMask=1  BitMaskRealWorld=Stored Integer
      settings: LibrarySourceBlock=|
      | simulink/Quick Insert/Logic and Bit
      | Operations/Bitwise AND
  Bitwise AND1 : simulink/Logic and Bit Operations/Bitwise Operator  logicop=AND  UseBitMask=on  BitMask=2  BitMaskRealWorld=Stored Integer
      settings: LibrarySourceBlock=|
      | simulink/Quick Insert/Logic and Bit
      | Operations/Bitwise AND
  Bitwise AND2 : simulink/Logic and Bit Operations/Bitwise Operator  logicop=AND  UseBitMask=on  BitMask=4  BitMaskRealWorld=Stored Integer
      settings: LibrarySourceBlock=|
      | simulink/Quick Insert/Logic and Bit
      | Operations/Bitwise AND
  Bitwise AND3 : simulink/Logic and Bit Operations/Bitwise Operator  logicop=AND  UseBitMask=on  BitMask=8  BitMaskRealWorld=Stored Integer
      settings: LibrarySourceBlock=|
      | simulink/Quick Insert/Logic and Bit
      | Operations/Bitwise AND
  Bitwise AND4 : simulink/Logic and Bit Operations/Bitwise Operator  logicop=AND  UseBitMask=on  BitMask=16  BitMaskRealWorld=Stored Integer
      settings: LibrarySourceBlock=|
      | simulink/Quick Insert/Logic and Bit
      | Operations/Bitwise AND
  Bitwise OR : simulink/Logic and Bit Operations/Bitwise Operator  logicop=OR  UseBitMask=off  NumInputPorts=3  BitMask=bin2dec('11011001')  BitMaskRealWorld=Stored Integer
      settings: LibrarySourceBlock=|
      | simulink/Quick Insert/Logic and Bit
      | Operations/Bitwise OR
  Constant : Constant
  Constant1 : Constant
  Constant2 : Constant
  OR : Logic  Operator=OR  Inputs=3  AllPortsSameDT=off  OutDataTypeStr=boolean
  OV and UV fault : Subsystem
  Selector : Selector  InputPortWidth=3  IndexOptions=Index vector (dialog)  Indices=1  OutputSizes=1
  Selector1 : Selector  InputPortWidth=3  IndexOptions=Index vector (dialog)  Indices=2  OutputSizes=1
  Selector2 : Selector  InputPortWidth=3  IndexOptions=Index vector (dialog)  Indices=3  OutputSizes=1
  Subsystem : Subsystem
  Vector Concatenate1 : Concatenate  NumInputs=3
  Vector Concatenate2 : Concatenate  NumInputs=5
  FAULT : Outport
  FAULT_SUM : Outport  Port=2
  FaultPlace : Outport  Port=3
  wires:
  Subsystem/3(AUX2_OV_FAULT) -> Vector Concatenate2/3
  [UV_FAULT_SUM] -> Bit Shift/1
  [UV_FAULT_SUM] -> OR/1
  [Latch] -> Subsystem/11(LatchAUX3_OV)
  [OV_FAULT_SUM] -> Bit Shift1/1
  [OV_FAULT_SUM] -> OR/2
  Subsystem/1(AUX0_OV_FAULT) -> Vector Concatenate2/1
  [Latch] -> Subsystem/13(LatchAUX4_OV)
  Subsystem/4(AUX3_OV_FAULT) -> Vector Concatenate2/4
  OV and UV fault/4(OV_FAULT) -> [FAULT_OV]
  OR/1 -> FAULT/1
  OV and UV fault/3(OV_FAULT _SUM) -> [OV_FAULT_SUM]
  [AUXOV_FAULT_SUM] -> Bit Shift2/1
  [AUXOV_FAULT_SUM] -> OR/3
  [ResetOV] -> OV and UV fault/5(ResetOV)
  OV and UV fault/1(UV_FAULT _SUM) -> [UV_FAULT_SUM]
  Bitwise AND3/1 -> Subsystem/12(ResetAUX3_OV)
  [Latch] -> Subsystem/9(LatchAUX2_OV)
  Subsystem/5(AUX4_OV_FAULT) -> Vector Concatenate2/5
  OV and UV fault/2(UV_FAULT) -> [FAULT_UV]
  Subsystem/6(AUXOV_FAULT_SUM) -> [AUXOV_FAULT_SUM]
  Bitwise AND/1 -> Subsystem/3(ResetAUX0_OV)
  Vector Concatenate1/1 -> FaultPlace/1
  Bitwise AND2/1 -> Subsystem/10(ResetAUX2_OV)
  [ResetUV] -> OV and UV fault/3(ResetUV)
  [FAULT_OV] -> Vector Concatenate1/2
  Bitwise OR/1 -> FAULT_SUM/1
  [Latch] -> OV and UV fault/4(LatchOV)
  [FAULT_UV] -> Vector Concatenate1/1
  [Latch] -> Subsystem/2(LatchAUX0_OV)
  Subsystem/2(AUX1_OV_FAULT) -> Vector Concatenate2/2
  [Latch] -> Subsystem/4(LatchAUX1_OV)
  Bitwise AND1/1 -> Subsystem/5(ResetAUX1_OV)
  CellVoltages/1 -> OV and UV fault/1(CellVoltages)
  ModuleCurrent/1 -> Subsystem/1(ModuleCurrent)
  UNLATCH/1 -> [Latch]
  [Latch] -> OV and UV fault/2(LatchUV)
  Selector/1 -> [ResetUV]
  Selector1/1 -> [ResetOV]
  Constant/1 -> Subsystem/6(TemperatureSensor1)  "Temp1"
  Constant1/1 -> Subsystem/7(TemperatureSensor2)  "Temp2"
  Constant2/1 -> Subsystem/8(TemperatureSensor3)  "Temp3"
  Reset/1 -> Selector1/1, Selector/1, Selector2/1
  Bitwise AND4/1 -> Subsystem/14(ResetAUX4_OV)
  Vector Concatenate2/1 -> Bit to Integer Converter/1
  Bit to Integer Converter/1 -> [FAULT_AUX]
  [FAULT_AUX] -> Vector Concatenate1/3
  Bit Shift1/1 -> Bitwise OR/2
  Bit Shift2/1 -> Bitwise OR/3
  Bit Shift/1 -> Bitwise OR/1
  Selector2/1 -> Bitwise AND/1, Bitwise AND2/1, Bitwise AND3/1, Bitwise AND4/1, Bitwise AND1/1
